simulink model "adcs_v14_speed"  (Simulink 7.4)
settings: Solver=ode4  StartTime=0.0  StopTime=80000  FixedStep=s_SIM_STEP_SIZE  RelTol=1e-3
values from neighbouring files (symbols this model uses):
  A = ((T_SIDE + .29)*1e-3)^2    [constants_v13.m]    (also in constants_v15.m; constants_v15_Pow.m; constants_v15_Pow_ss_error.m; constants_v16_integral_kartavya.m)
  Ca_Solar_Drag = 1.4    [constants_v13.m]    (also in constants_v15.m = 0; constants_v15_Pow.m; constants_v15_Pow_ss_error.m; constants_v16_integral_kartavya.m)
  Cd = 2.2    [constants_v13.m]    (also in constants_v15.m = 0; constants_v15_Pow.m; constants_v15_Pow_ss_error.m; constants_v16_integral_kartavya.m)
  check_time = 60000    [constants_v13.m]    (also in constants_v15.m = 10000; constants_v15_Pow_ss_error.m = 10000; constants_v16_integral_kartavya.m = 10000; constants_v16_integral_light_sun_sgp_igrf_power_13Dec2011.m = 10000)
  I_MAX = 0.5    [constants_v13.m]    (also in constants_v15.m; constants_v15_Pow.m; constants_v15_Pow_ss_error.m; constants_v16_integral_kartavya.m)
  I_TORQUER = 3.6 / 7.31    (= 0.492476060192)    [constants_v13.m]    (also in constants_v15.m = 0.272727272727; constants_v15_Pow.m; constants_v15_Pow_ss_error.m; constants_v16_integral_kartavya.m)
  Kd = 2* m_INERTIA / (s_numOrbits * T_ORBIT )    [constants_v13.m]    (also in constants_v15.m = m_INERTIA * (2 + delta)* zeta * w; constants_v15_Pow.m = m_INERTIA * (2 + delta)* zeta * w; constants_v15_Pow_ss_error.m = m_INERTIA * (2 + delta)* zeta * w; constants_v16_integral_kartavya.m = m_INERTIA * (2 + delta)* zeta * w)
  Kdetumb = K_det*eye(3)    [constants_v13.m]    (also in constants_v15.m; constants_v15_Pow.m; constants_v15_Pow_ss_error.m; constants_v16_integral_kartavya.m)
  Kp = m_INERTIA / (s_numOrbits * T_ORBIT * zeta)^2    [constants_v13.m]    (also in constants_v15.m = m_INERTIA * (w*w + 2*delta*zeta^2*w^2); constants_v15_Pow.m = m_INERTIA * (w*w + 2*delta*zeta^2*w^2); constants_v15_Pow_ss_error.m = m_INERTIA * (w*w + 2*delta*zeta^2*w^2); constants_v16_integral_kartavya.m = m_INERTIA * (w*w + 2*delta*zeta^2*w^2))
  m_INERTIA = [Ixx Ixy Ixz; Ixy Iyy Iyz; Ixz Iyz Izz]    [constants_v13.m]    (also in constants_v15.m; constants_v15_Pow.m = 1*[Ixx Ixy Ixz; Ixy Iyy Iyz; Ixz Iyz Izz]; constants_v15_Pow_ss_error.m = 1*[Ixx Ixy Ixz; Ixy Iyy Iyz; Ixz Iyz Izz]; constants_v16_integral_kartavya.m)
  mu = 6.673e-11*5.9742e24    (= 398658366000000)    [constants_v13.m]    (also in constants_v15.m; constants_v15_Pow.m; constants_v15_Pow_ss_error.m; constants_v16_integral_kartavya.m)
  N = 40    [constants_v13.m]    (also in constants_v15.m = 60; constants_v15_Pow.m; constants_v15_Pow_ss_error.m; constants_v16_integral_kartavya.m)
  P_momentum_flux_from_the_sun = 4.4e-6    (= 4.4e-06)    [constants_v13.m]    (also in constants_v15.m = 0; constants_v15_Pow.m; constants_v15_Pow_ss_error.m; constants_v16_integral_kartavya.m)
  q_BI0 = x_fromEnvModel(1:4)'    [OILS_script.m]    (also in OILS_script_OBC_preflight_bounce_back.m; OILS_script_extended.m; OILS_script_preflight_test.m; constants_v13.m = euler2qBI(roll0,pitch0,yaw0))
  s_FRAME_SIZE = 2    [constants_v13.m]    (also in constants_v15.m; constants_v15_Pow.m; constants_v15_Pow_ss_error.m; constants_v16_integral_kartavya.m)
  s_m_MAX = 0.95    [constants_v13.m]    (also in constants_v15.m; constants_v15_Pow.m; constants_v15_Pow_ss_error.m; constants_v16_integral_kartavya.m)
  s_MAG_B = 2.5e-5    (= 2.5e-05)    [constants_v13.m]    (also in constants_v15.m; constants_v15_Pow.m; constants_v15_Pow_ss_error.m; constants_v16_integral_kartavya.m)
  s_MAGMETER_WEIGHT = .9    (= 0.9)    [constants_v13.m]    (also in constants_v15.m; constants_v15_Pow.m; constants_v15_Pow_ss_error.m; constants_v16_integral_kartavya.m)
  s_SIM_STEP_SIZE = 0.1    [constants_v13.m]    (also in constants_v15.m; constants_v15_Pow.m; constants_v15_Pow_ss_error.m; constants_v16_integral_kartavya.m)
  s_SS_ADC_gain = 5    [constants_v13.m]    (also in constants_v15.m = 3.3; constants_v15_Pow.m; constants_v15_Pow_ss_error.m; constants_v16_integral_kartavya.m)
  s_SS_ADC_res = 2^12 - 1    (= 4095)    [constants_v13.m]    (also in constants_v15.m = 1023; constants_v15_Pow.m; constants_v15_Pow_ss_error.m; constants_v16_integral_kartavya.m)
  s_SS_MAX_ANGLE = 85    [constants_v13.m]    (also in constants_v15.m = 55; constants_v15_Pow.m; constants_v15_Pow_ss_error.m; constants_v16_integral_kartavya.m)
  s_TAU_W = 60    [constants_v13.m]    (also in constants_v15.m; constants_v15_Pow.m; constants_v15_Pow_ss_error.m; constants_v16_integral_kartavya.m)
  s_x_MAGMETER_BIAS = 50e-9    (= 5e-08)    [constants_v13.m]    (also in constants_v15.m = 0; constants_v15_Pow.m; constants_v15_Pow_ss_error.m; constants_v16_integral_kartavya.m)
  side = 0.26    [constants_v13.m]    (also in constants_v15.m; constants_v15_Pow.m; constants_v15_Pow_ss_error.m; constants_v16_integral_kartavya.m)
  Snum = 6    [constants_v13.m]    (also in constants_v15.m; constants_v15_Pow.m; constants_v15_Pow_ss_error.m; constants_v16_integral_kartavya.m)
  tol_q4 = 0.7    [constants_v13.m]    (also in constants_v15.m = 0.85; constants_v15_Pow.m = 0.85; constants_v15_Pow_ss_error.m = 0.85; constants_v16_integral_kartavya.m = 0.85)
  tol_w = 4e-3    (= 0.004)    [constants_v13.m]    (also in constants_v15.m; constants_v15_Pow.m; constants_v15_Pow_ss_error.m; constants_v16_integral_kartavya.m)
  Ts_display = 6    [constants_v13.m]    (also in constants_v15.m = 2; constants_v15_Pow.m; constants_v15_Pow_ss_error.m; constants_v16_integral_kartavya.m)
  v_COM_to_COP_b = [.2; 1.75; .2]*1e-2    [constants_v13.m]    (also in constants_v15.m = [.2; 1.75; .2]*0e-2; constants_v15_Pow.m; constants_v15_Pow_ss_error.m; constants_v16_integral_kartavya.m)
  v_S1 = [1 0 0]    [constants_v13.m]    (also in constants_v15.m; constants_v15_Pow.m; constants_v15_Pow_ss_error.m; constants_v16_integral_kartavya.m)
  v_S2 = [-1 0 0]    [constants_v13.m]    (also in constants_v15.m; constants_v15_Pow.m; constants_v15_Pow_ss_error.m; constants_v16_integral_kartavya.m)
  v_S3 = [0 1 0]    [constants_v13.m]    (also in constants_v15.m; constants_v15_Pow.m; constants_v15_Pow_ss_error.m; constants_v16_integral_kartavya.m)
  v_S4 = [0 -1 0]    [constants_v13.m]    (also in constants_v15.m; constants_v15_Pow.m; constants_v15_Pow_ss_error.m; constants_v16_integral_kartavya.m)
  v_S5 = [0 0 1]    [constants_v13.m]    (also in constants_v15.m; constants_v15_Pow.m; constants_v15_Pow_ss_error.m; constants_v16_integral_kartavya.m)
  v_S6 = [0 0 -1]    [constants_v13.m]    (also in constants_v15.m; constants_v15_Pow.m; constants_v15_Pow_ss_error.m; constants_v16_integral_kartavya.m)
  v_x_MOUNTING_THETA_ZYX_BODY_TORQUER = [1; 1; 1]* pi/180    [constants_v13.m]    (also in constants_v15.m; constants_v15_Pow.m; constants_v15_Pow_ss_error.m; constants_v16_integral_kartavya.m)
  wx0 = x_fromEnvModel(5)    [OILS_script.m]    (also in OILS_script_OBC_preflight_bounce_back.m; OILS_script_extended.m; OILS_script_preflight_test.m; constants_v13.m = 0.0349065850399)
  wy0 = x_fromEnvModel(6)    [OILS_script.m]    (also in OILS_script_OBC_preflight_bounce_back.m; OILS_script_extended.m; OILS_script_preflight_test.m; constants_v13.m = 0.0174532925199)
  wz0 = x_fromEnvModel(7)    [OILS_script.m]    (also in OILS_script_OBC_preflight_bounce_back.m; OILS_script_extended.m; OILS_script_preflight_test.m; constants_v13.m = -0.0349065850399)
libraries: commnoisgen2 x7, simulink x4, aerolibutil x2
(part 1 of 2)
settings Model: Creator=Jaideep  LastModifiedBy=Jaideep  SimulationMode=rapid-accelerator  ExtModeTrigDuration=100
settings SolverCC: AutoInsertRateTranBlk=on
settings DataIOCC: SaveFinalState=on  SaveOutput=off  SaveState=on  StateSaveName=tmp_raccel_xout
settings OptimizationCC: EfficientMapNaN2IntZero=off
settings HardwareCC: TargetEndianess=LittleEndian  TargetHWDeviceType=MATLAB Host  ProdEqTarget=off
settings RTWCC: SystemTargetFile=raccel.tlc  TemplateMakefile=raccel_default_tmf  RTWVerbose=off  ProcessScript=raccel_make_rtw_hook
settings CodeAppCC: GenerateComments=off  MaxIdLength=128  SimulinkBlockComments=off
settings RaccelTargetCC: TargetFunctionLibrary=ANSI_C  ERTMultiwordTypeDef=System defined  ERTMultiwordLength=256  IsPILTarget=off  ParMdlRefBuildCompliant=off  GeneratePreprocessorConditionals=Disable all  ERTFirstTimeCompliant=off  MultiInstanceERTCode=off  EnableShiftOperators=on  PortableWordSizes=off  RTWCAPISignals=off  RTWCAPIParams=off

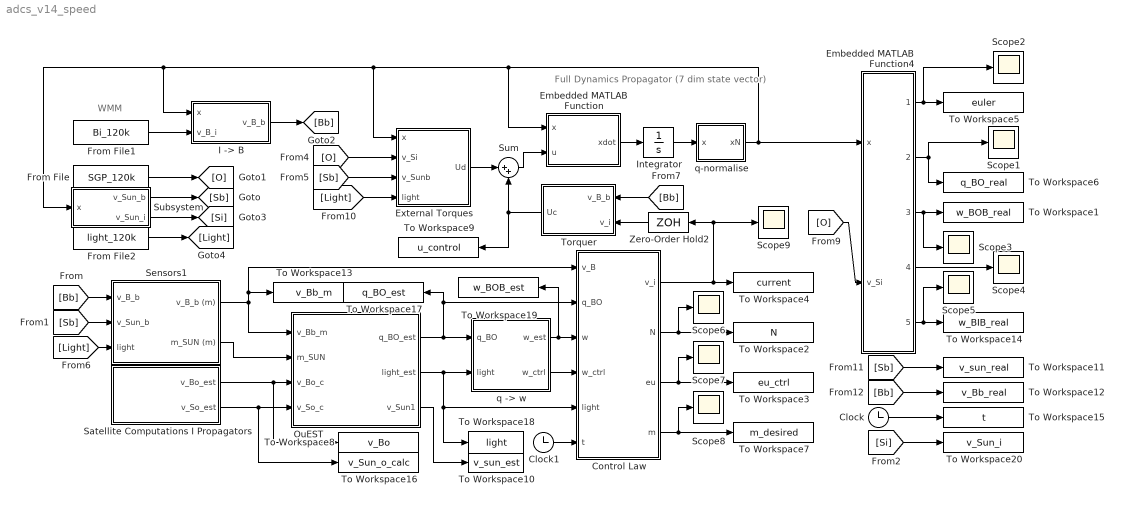
== system adcs_v14_speed ==
  note: Full Dynamics Propagator
      |  (7 dim state vector)
  note: WMM
  Clock : Clock
      settings: Decimation=10
  Clock1 : Clock
      settings: Decimation=10
  Control Law : Subsystem  TreatAsAtomicUnit=on  SystemSampleTime=s_FRAME_SIZE
  Embedded MATLAB Function : Stateflow chart
  Embedded MATLAB Function4 : Stateflow chart
  External Torques : Subsystem
  From File : FromFile  FileName=SGP_120k
  From File1 : FromFile  FileName=Bi_120k
  From File2 : FromFile  FileName=light_120k  SampleTime=0
  "I -> B" : Subsystem
  Integrator : Integrator  InitialCondition=[q_BI0; wx0; wy0; wz0]
  QuEST : Stateflow chart  TreatAsAtomicUnit=on  SystemSampleTime=s_FRAME_SIZE
  Satellite Computations I Propagators : Subsystem  TreatAsAtomicUnit=on  SystemSampleTime=s_FRAME_SIZE
  Scope{1..9} (9 alike) : Scope
      Scope1 settings: YMin=-10  YMax=10  SaveName=ScopeData11  SampleInput=on  SampleTime=Ts_display
      Scope2 settings: TimeRange=80000  YMin=-70  YMax=60  SaveName=ScopeData7  SampleInput=on  SampleTime=Ts_display
      Scope3 settings: YMin=-10  YMax=10  SaveName=ScopeData13  SampleInput=on  SampleTime=Ts_display
      Scope4 settings: YMin=-10  YMax=10  SaveName=ScopeData14  SampleInput=on  SampleTime=Ts_display
      Scope5 settings: YMin=-10  YMax=10  SaveName=ScopeData15  SampleInput=on  SampleTime=Ts_display
      Scope6 settings: YMin=-10  YMax=10  SaveName=ScopeData16  SampleInput=on  SampleTime=Ts_display
      Scope7 settings: YMin=-10  YMax=10  SaveName=ScopeData20  SampleInput=on  SampleTime=Ts_display
      Scope8 settings: YMin=-10  YMax=10  SaveName=ScopeData21  SampleInput=on  SampleTime=Ts_display
      Scope9 settings: YMin=-10  YMax=10  SaveName=ScopeData23  SampleInput=on  SampleTime=Ts_display
  Sensors1 : Subsystem
  Subsystem : Subsystem
  Sum : Sum  Inputs=|++  OutDataType=sfix(16)  OutScaling=2^0
  To Workspace1 : ToWorkspace  VariableName=w_BOB_real  SampleTime=Ts_display  SaveFormat=Array
  To Workspace10 : ToWorkspace  VariableName=v_sun_est  SampleTime=Ts_display  SaveFormat=Array
  To Workspace11 : ToWorkspace  VariableName=v_sun_real  SampleTime=Ts_display  SaveFormat=Array
  To Workspace12 : ToWorkspace  VariableName=v_Bb_real  SampleTime=Ts_display  SaveFormat=Array
  To Workspace13 : ToWorkspace  VariableName=v_Bb_m  SampleTime=Ts_display  SaveFormat=Array
  To Workspace14 : ToWorkspace  VariableName=w_BIB_real  SampleTime=Ts_display  SaveFormat=Array
  To Workspace15 : ToWorkspace  VariableName=t  SampleTime=Ts_display  SaveFormat=Array
  To Workspace16 : ToWorkspace  VariableName=v_Sun_o_calc  SampleTime=Ts_display  SaveFormat=Array
  To Workspace17 : ToWorkspace  VariableName=q_BO_est  SampleTime=Ts_display  SaveFormat=Array
  To Workspace18 : ToWorkspace  VariableName=light  SampleTime=Ts_display  SaveFormat=Array
  To Workspace19 : ToWorkspace  VariableName=w_BOB_est  SampleTime=Ts_display  SaveFormat=Array
  To Workspace2 : ToWorkspace  VariableName=N  SampleTime=Ts_display  SaveFormat=Array
  To Workspace20 : ToWorkspace  VariableName=v_Sun_i  SampleTime=Ts_display  SaveFormat=Array
  To Workspace3 : ToWorkspace  VariableName=eu_ctrl  SampleTime=Ts_display  SaveFormat=Array
  To Workspace4 : ToWorkspace  VariableName=current  SampleTime=Ts_display  SaveFormat=Array
  To Workspace5 : ToWorkspace  VariableName=euler  SampleTime=Ts_display  SaveFormat=Array
  To Workspace6 : ToWorkspace  VariableName=q_BO_real  SampleTime=Ts_display  SaveFormat=Array
  To Workspace7 : ToWorkspace  VariableName=m_desired  SampleTime=Ts_display  SaveFormat=Array
  To Workspace8 : ToWorkspace  VariableName=v_Bo  SampleTime=Ts_display  SaveFormat=Array
  To Workspace9 : ToWorkspace  VariableName=u_control  SampleTime=Ts_display  SaveFormat=Array
  Torquer : Subsystem
  Zero-Order Hold2 : ZeroOrderHold  SampleTime=s_FRAME_SIZE
  "q -> w" : Subsystem  TreatAsAtomicUnit=on  SystemSampleTime=s_FRAME_SIZE
  q-normalise : Stateflow chart
  wires:
  Embedded MATLAB Function/1(xdot) -> Integrator/1
  Integrator/1 -> q-normalise/1(x)
  From File/1 -> [O]
  q-normalise/1(xN) -> Subsystem/1(x), "I -> B"/1(x), External Torques/1(x), Embedded MATLAB Function/1(x), Embedded MATLAB Function4/1(x)
  Sum/1 -> Embedded MATLAB Function/2(u)
  "I -> B"/1(v_B_b) -> [Bb]
  Subsystem/1(v_Sun_b) -> [Sb]
  [Bb] -> Sensors1/1(v_B_b)
  [Sb] -> Sensors1/2(v_Sun_b)
  Subsystem/2(v_Sun_i) -> [Si]
  [O] -> External Torques/2(v_Si)
  [Sb] -> External Torques/3(v_Sunb)
  [Bb] -> Torquer/1(v_B_b)
  [Light] -> Sensors1/3(light)
  Sensors1/2(m_SUN (m)) -> QuEST/2(m_SUN)
  Sensors1/1(v_B_b (m)) -> QuEST/1(v_Bb_m), Control Law/1(v_B), To Workspace13/1
  Zero-Order Hold2/1 -> Torquer/2(v_i)
  External Torques/1(Ud) -> Sum/1
  Torquer/1(Uc) -> Sum/2, To Workspace9/1
  Satellite Computations I Propagators/1(v_Bo_est) -> To Workspace8/1, QuEST/3(v_Bo_c)
  Satellite Computations I Propagators/2(v_So_est) -> To Workspace16/1, QuEST/4(v_So_c)
  QuEST/1(q_BO_est) -> "q -> w"/1(q_BO), Control Law/2(q_BO), To Workspace17/1
  QuEST/2(light_est) -> "q -> w"/2(light), Control Law/5(light), To Workspace18/1
  Control Law/1(v_i) -> To Workspace4/1, Zero-Order Hold2/1, Scope9/1
  [O] -> Embedded MATLAB Function4/2(v_Si)
  Control Law/2(N) -> To Workspace2/1, Scope6/1
  From File2/1 -> [Light]
  Control Law/3(eu) -> To Workspace3/1, Scope7/1
  Control Law/4(m) -> To Workspace7/1, Scope8/1
  "q -> w"/1(w_est) -> Control Law/3(w), To Workspace19/1
  [Light] -> External Torques/4(light)
  "q -> w"/2(w_ctrl) -> Control Law/4(w_ctrl)
  QuEST/3(v_Sun1) -> To Workspace10/1
  [Sb] -> To Workspace11/1
  [Bb] -> To Workspace12/1
  Clock/1 -> To Workspace15/1
  From File1/1 -> "I -> B"/2(v_B_i)
  Clock1/1 -> Control Law/6(t)
  Embedded MATLAB Function4/3(w_BOB) -> To Workspace1/1, Scope3/1
  Embedded MATLAB Function4/2(q_BO) -> To Workspace6/1, Scope1/1
  Embedded MATLAB Function4/1(euler) -> To Workspace5/1, Scope2/1
  Embedded MATLAB Function4/5(w_BIB) -> To Workspace14/1, Scope5/1
  Embedded MATLAB Function4/4(modw) -> Scope4/1
  [Si] -> To Workspace20/1

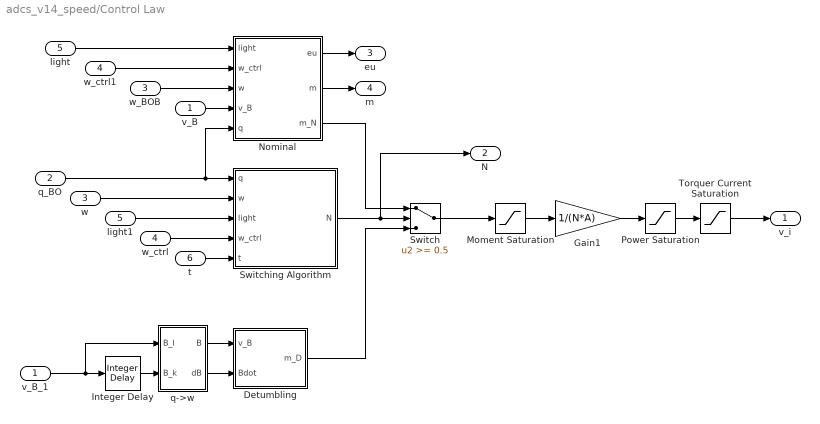
== system adcs_v14_speed/Control Law ==
  v_B : Inport  OutDataType=sfix(16)  OutScaling=2^0
  q_BO : Inport  Port=2  OutDataType=sfix(16)  OutScaling=2^0
  w : Inport  Port=3  OutDataType=sfix(16)  OutScaling=2^0
  w_ctrl : Inport  Port=4  OutDataType=sfix(16)  OutScaling=2^0
  light : Inport  Port=5  OutDataType=sfix(16)  OutScaling=2^0
  t : Inport  Port=6  OutDataType=sfix(16)  OutScaling=2^0
  Detumbling : Stateflow chart
  Gain1 : Gain  Gain=1/(N*A)  ParameterDataType=sfix(16)  ParameterScaling=2^0  OutDataType=sfix(16)  OutScaling=2^0
  Integer Delay : simulink/Discrete/Integer Delay  vinit=0.0  samptime=-1  NumDelays=1
  Moment Saturation : Saturate  UpperLimit=s_m_MAX  LowerLimit=-s_m_MAX  OutDataType=sfix(16)  OutScaling=2^0
  Nominal : Stateflow chart
  Power Saturation : Saturate  UpperLimit=I_MAX  LowerLimit=-I_MAX  OutDataType=sfix(16)  OutScaling=2^0
  Switch : Switch  Threshold=0.5  OutDataType=sfix(16)  OutScaling=2^0
  Switching Algorithm : Subsystem
  Torquer Current Saturation : Saturate  UpperLimit=I_TORQUER  LowerLimit=-I_TORQUER  OutDataType=sfix(16)  OutScaling=2^0
  light1 : InportShadow  Port=5  OutDataType=sfix(16)  OutScaling=2^0  LatchByCopyingInsideSignal=off
  q->w : Stateflow chart
  v_B_1 : InportShadow  Port=1  OutDataType=sfix(16)  OutScaling=2^0  LatchByCopyingInsideSignal=off
  w_BOB : InportShadow  Port=3  OutDataType=sfix(16)  OutScaling=2^0  LatchByCopyingInsideSignal=off
  w_ctrl1 : InportShadow  Port=4  OutDataType=sfix(16)  OutScaling=2^0  LatchByCopyingInsideSignal=off
  v_i : Outport  OutDataType=sfix(16)  OutScaling=2^0
  N : Outport  Port=2  OutDataType=sfix(16)  OutScaling=2^0
  eu : Outport  Port=3  OutDataType=sfix(16)  OutScaling=2^0
  m : Outport  Port=4  OutDataType=sfix(16)  OutScaling=2^0
  wires:
  w_ctrl/1 -> Switching Algorithm/4(w_ctrl)
  Nominal/2(m) -> m/1
  Nominal/1(eu) -> eu/1
  w_BOB/1 -> Nominal/3(w)
  light1/1 -> Switching Algorithm/3(light)
  v_B/1 -> Nominal/4(v_B)
  q->w/2(dB) -> Detumbling/2(Bdot)
  v_B_1/1 -> Integer Delay/1, q->w/1(B_l)
  w/1 -> Switching Algorithm/2(w)
  Nominal/3(m_N) -> Switch/1
  Switching Algorithm/1(N) -> Switch/2, N/1
  Detumbling/1(m_D) -> Switch/3
  Switch/1 -> Moment Saturation/1
  Power Saturation/1 -> Torquer Current Saturation/1
  Moment Saturation/1 -> Gain1/1
  Torquer Current Saturation/1 -> v_i/1
  Gain1/1 -> Power Saturation/1
  light/1 -> Nominal/1(light)
  q_BO/1 -> Switching Algorithm/1(q), Nominal/5(q)
  Integer Delay/1 -> q->w/2(B_k)
  q->w/1(B) -> Detumbling/1(v_B)
  t/1 -> Switching Algorithm/5(t)
  w_ctrl1/1 -> Nominal/2(w_ctrl)

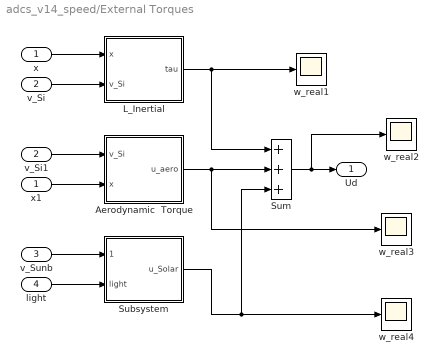
== system adcs_v14_speed/External Torques ==
  x : Inport  OutDataType=sfix(16)  OutScaling=2^0
  v_Si : Inport  Port=2  OutDataType=sfix(16)  OutScaling=2^0
  v_Sunb : Inport  Port=3  OutDataType=sfix(16)  OutScaling=2^0
  light : Inport  Port=4  OutDataType=sfix(16)  OutScaling=2^0
  Aerodynamic  Torque : Subsystem
  L_Inertial : Stateflow chart
  Subsystem : Subsystem
  Sum : Sum  Inputs=+++  OutDataType=fixdt(1, 16)  OutScaling=2^0
  v_Si1 : InportShadow  Port=2  OutDataType=sfix(16)  OutScaling=2^0  LatchByCopyingInsideSignal=off
  w_real{1..4} (4 alike) : Scope
      w_real1 settings: TimeRange=80000  YMin=-3e-009  YMax=1.1e-008  SaveName=ScopeData18  SampleInput=on  SampleTime=5
      w_real2 settings: TimeRange=80000  YMin=-7e-009  YMax=1e-008  SaveName=ScopeData17  SampleInput=on  SampleTime=5
      w_real3 settings: YMin=-8e-010  YMax=1.4e-009  SaveName=ScopeData19  SampleInput=on  SampleTime=5
      w_real4 settings: YMin=-6e-009  YMax=1e-008  SaveName=ScopeData22  SampleInput=on  SampleTime=5
  x1 : InportShadow  Port=1  OutDataType=sfix(16)  OutScaling=2^0  LatchByCopyingInsideSignal=off
  Ud : Outport  OutDataType=sfix(16)  OutScaling=2^0
  wires:
  x/1 -> L_Inertial/1(x)
  v_Si/1 -> L_Inertial/2(v_Si)
  L_Inertial/1(tau) -> Sum/1, w_real1/1
  Aerodynamic  Torque/1(u_aero) -> Sum/2, w_real3/1
  x1/1 -> Aerodynamic  Torque/2(x)
  v_Si1/1 -> Aerodynamic  Torque/1(v_Si)
  Sum/1 -> Ud/1, w_real2/1
  v_Sunb/1 -> Subsystem/1(v_Sun_b)
  Subsystem/1(u_Solar) -> Sum/3, w_real4/1
  light/1 -> Subsystem/2(light)

== system adcs_v14_speed/I -> B ==
  x : Inport  OutDataType=sfix(16)  OutScaling=2^0
  v_B_i : Inport  Port=2  OutDataType=sfix(16)  OutScaling=2^0
  Gain : Gain  Gain=1e-9  ParameterDataType=fixdt(1, 16)  ParameterScaling=2^0  OutDataType=fixdt(1, 16)  OutScaling=2^0
  L_Inertial : Stateflow chart
  v_B_b : Outport  OutDataType=sfix(16)  OutScaling=2^0
  wires:
  L_Inertial/1(v_B) -> v_B_b/1
  x/1 -> L_Inertial/1(x)
  v_B_i/1 -> Gain/1
  Gain/1 -> L_Inertial/2(v_I)

== system adcs_v14_speed/Satellite Computations I Propagators ==
  From File : FromFile  FileName=Si_120k
  From File2 : FromFile  FileName=SGP_est_120k
  From File3 : FromFile  FileName=Bi8_est_120k
  m_TOI_NEW : Stateflow chart
  m_TOI_NEW1 : Stateflow chart
  v_Bo_est : Outport  OutDataType=sfix(16)  OutScaling=2^0
  v_So_est : Outport  Port=2  OutDataType=sfix(16)  OutScaling=2^0
  wires:
  From File3/1 -> m_TOI_NEW/2(v_I)
  From File2/1 -> m_TOI_NEW1/2(ECI), m_TOI_NEW/1(ECI)
  From File/1 -> m_TOI_NEW1/1(v_I)
  m_TOI_NEW/1(v_O) -> v_Bo_est/1
  m_TOI_NEW1/1(v_O) -> v_So_est/1

== system adcs_v14_speed/Sensors1 ==
  note: 'm' stands for measured
  v_B_b : Inport  OutDataType=sfix(16)  OutScaling=2^0
  v_Sun_b : Inport  Port=2  OutDataType=sfix(16)  OutScaling=2^0
  light : Inport  Port=3  OutDataType=sfix(16)  OutScaling=2^0
  Magnetometer simple : Subsystem
  Sun Sensors : Subsystem
  v_B_b (m) : Outport  OutDataType=sfix(16)  OutScaling=2^0
  m_SUN (m) : Outport  Port=2  OutDataType=sfix(16)  OutScaling=2^0
  wires:
  light/1 -> Sun Sensors/2(Light)
  Magnetometer simple/1(v_B_b(m)) -> v_B_b (m)/1
  v_B_b/1 -> Magnetometer simple/1(v_B_b)
  v_Sun_b/1 -> Sun Sensors/1(v_Sun_b)
  Sun Sensors/1(m_SUN) -> m_SUN (m)/1

== system adcs_v14_speed/Subsystem ==
  x : Inport  OutDataType=sfix(16)  OutScaling=2^0
  From File : FromFile  FileName=Si_120k  SampleTime=0
  f: I->B : Stateflow chart
  v_Sun_b : Outport  OutDataType=sfix(16)  OutScaling=2^0
  v_Sun_i : Outport  Port=2  OutDataType=sfix(16)  OutScaling=2^0
  wires:
  x/1 -> f: I->B/1(x)
  f: I->B/1(v_B) -> v_Sun_b/1
  From File/1 -> f: I->B/2(v_I), v_Sun_i/1

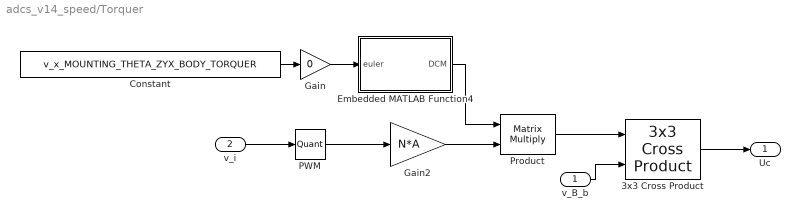
== system adcs_v14_speed/Torquer ==
  v_B_b : Inport  OutDataType=sfix(16)  OutScaling=2^0
  v_i : Inport  Port=2  OutDataType=sfix(16)  OutScaling=2^0
  3x3 Cross Product : aerolibutil/3x3 Cross Product  SystemSampleTime=-1
  Constant : Constant  Value=v_x_MOUNTING_THETA_ZYX_BODY_TORQUER  OutDataType=sfix(16)  OutScaling=2^0
  Embedded MATLAB Function4 : Stateflow chart
  Gain : Gain  Gain=0  ParameterDataType=sfix(16)  ParameterScaling=2^0  OutDataType=sfix(16)  OutScaling=2^0
  Gain2 : Gain  Gain=N*A  ParameterDataType=sfix(16)  ParameterScaling=2^0  OutDataType=sfix(16)  OutScaling=2^0
  PWM : Quantizer  QuantizationInterval=s_PWM_RES
  Product : Product  Multiplication=Matrix(*)  OutDataType=sfix(16)  OutScaling=2^0  RndMeth=Zero
  Uc : Outport  OutDataType=sfix(16)  OutScaling=2^0
  wires:
  PWM/1 -> Gain2/1
  v_B_b/1 -> 3x3 Cross Product/2
  3x3 Cross Product/1 -> Uc/1
  v_i/1 -> PWM/1
  Embedded MATLAB Function4/1(DCM) -> Product/1
  Gain2/1 -> Product/2
  Product/1 -> 3x3 Cross Product/1
  Constant/1 -> Gain/1
  Gain/1 -> Embedded MATLAB Function4/1(euler)

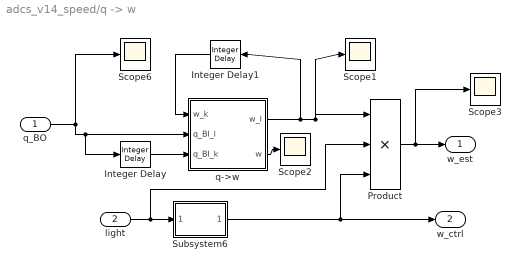
== system adcs_v14_speed/q -> w ==
  q_BO : Inport
  light : Inport  Port=2
  Integer Delay : simulink/Discrete/Integer Delay  vinit=0.0  samptime=-1  NumDelays=1
  Integer Delay1 : simulink/Discrete/Integer Delay  vinit=[0;0;0]  samptime=-1  NumDelays=1
  Product : Product  Inputs=3  OutDataType=fixdt(1, 16)  OutScaling=2^0  RndMeth=Zero
  Scope{1..3,6} (4 alike) : Scope
      Scope1 settings: YMin=-10  YMax=10  SaveName=ScopeData9  SampleInput=on
      Scope2 settings: YMin=-10  YMax=10  SaveName=ScopeData10  SampleInput=on
      Scope3 settings: YMin=-10  YMax=10  SaveName=ScopeData12  SampleInput=on
      Scope6 settings: YMin=-10  YMax=10  SaveName=ScopeData8  SampleInput=on
  Subsystem6 : Subsystem
  q->w : Stateflow chart
  w_est : Outport
  w_ctrl : Outport  Port=2
  wires:
  Subsystem6/1(w-ctrl) -> w_ctrl/1, Product/3
  q_BO/1 -> Integer Delay/1, q->w/2(q_BI_l), Scope6/1
  light/1 -> Product/2, Subsystem6/1(light)
  Product/1 -> w_est/1, Scope3/1
  Integer Delay/1 -> q->w/3(q_BI_k)
  q->w/1(w_l) -> Integer Delay1/1, Product/1, Scope1/1
  Integer Delay1/1 -> q->w/1(w_k)
  q->w/2(w) -> Scope2/1

== system adcs_v14_speed/Control Law/Switching Algorithm ==
  note: remov the t=0 checking
      | code, not necessary
  q : Inport  OutDataType=sfix(16)  OutScaling=2^0
  w : Inport  Port=2  OutDataType=sfix(16)  OutScaling=2^0
  light : Inport  Port=3  OutDataType=sfix(16)  OutScaling=2^0
  w_ctrl : Inport  Port=4  OutDataType=sfix(16)  OutScaling=2^0
  t : Inport  Port=5  OutDataType=sfix(16)  OutScaling=2^0
  Unit Delay : UnitDelay  SampleTime=-1
  gate pulse : Stateflow chart
  N : Outport  OutDataType=sfix(16)  OutScaling=2^0
  wires:
  t/1 -> gate pulse/3(t)
  w_ctrl/1 -> gate pulse/5(w_ctrl)
  light/1 -> gate pulse/4(light_flag)
  gate pulse/1(N) -> N/1
  q/1 -> gate pulse/2(q)
  Unit Delay/1 -> gate pulse/6(time2)
  gate pulse/2(time1) -> Unit Delay/1
  w/1 -> gate pulse/1(w)

== system adcs_v14_speed/External Torques/Aerodynamic  Torque ==
  v_Si : Inport
  x : Inport  Port=2
  Demux : Demux  Outputs=2
  aero torque : Stateflow chart
  v_I to v_B : Stateflow chart
  u_aero : Outport  OutDataType=sfix(16)  OutScaling=2^0
  wires:
  v_I to v_B/1(v_B) -> aero torque/2(v_B)
  v_Si/1 -> Demux/1
  Demux/2 -> v_I to v_B/1(v_I)
  x/1 -> v_I to v_B/2(x)
  aero torque/1(u_aero) -> u_aero/1

== system adcs_v14_speed/External Torques/Subsystem ==
  v_Sun_b : Inport  OutDataType=sfix(16)  OutScaling=2^0
  light : Inport  Port=2  OutDataType=sfix(16)  OutScaling=2^0
  Solar_drag : Stateflow chart
  Vector from CoM to CoP_in Body frame (yet to be finalized)2 : Constant  Value=v_COM_to_COP_b  VectorParams1D=off  OutDataType=sfix(16)  OutScaling=2^0
  _ : aerolibutil/3x3 Cross Product  SystemSampleTime=-1
  u_Solar : Outport  OutDataType=sfix(16)  OutScaling=2^0
  wires:
  _/1 -> u_Solar/1
  v_Sun_b/1 -> Solar_drag/1(v_Sun_b)
  light/1 -> Solar_drag/2(light)
  Solar_drag/1(solar_drag) -> _/2
  Vector from CoM to CoP_in Body frame (yet to be finalized)2/1 -> _/1

== system adcs_v14_speed/Sensors1/Magnetometer simple ==
  v_B_b : Inport  OutDataType=sfix(16)  OutScaling=2^0
  Constant : Constant  Value=s_x_MAGMETER_BIAS  OutDataType=fixdt(1, 16)  OutScaling=2^0
  Gaussian Noise Generator : commnoisgen2/Gaussian Noise Generator  SystemSampleTime=-1  m=0  d=s_x_MAGMETER  s=41  Ts=s_SIM_STEP_SIZE  frameBased=off  sampPerFrame=1  orient=off  outDataType=double
  Sum1 : Sum  Inputs=+++  OutDataType=sfix(16)  OutScaling=2^0
  v_B_b(m) : Outport  OutDataType=sfix(16)  OutScaling=2^0
  wires:
  Constant/1 -> Sum1/3
  Sum1/1 -> v_B_b(m)/1
  Gaussian Noise Generator/1 -> Sum1/1
  v_B_b/1 -> Sum1/2

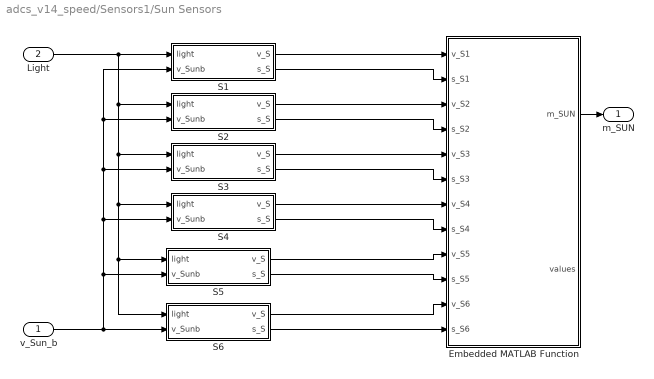
== system adcs_v14_speed/Sensors1/Sun Sensors ==
  v_Sun_b : Inport  OutDataType=sfix(16)  OutScaling=2^0
  Light : Inport  Port=2  OutDataType=sfix(16)  OutScaling=2^0
  Embedded MATLAB Function : Stateflow chart
  S1 : Subsystem
  S2 : Subsystem
  S3 : Subsystem
  S4 : Subsystem
  S5 : Subsystem
  S6 : Subsystem
  m_SUN : Outport  OutDataType=fixdt(1, 16)  OutScaling=2^0
  wires:
  Embedded MATLAB Function/1(m_SUN) -> m_SUN/1
  v_Sun_b/1 -> S6/2(v_Sunb), S5/2(v_Sunb), S4/2(v_Sunb), S3/2(v_Sunb), S2/2(v_Sunb), S1/2(v_Sunb)
  S1/1(v_S) -> Embedded MATLAB Function/1(v_S1)
  S1/2(s_S) -> Embedded MATLAB Function/2(s_S1)
  S2/1(v_S) -> Embedded MATLAB Function/3(v_S2)
  S2/2(s_S) -> Embedded MATLAB Function/4(s_S2)
  S3/1(v_S) -> Embedded MATLAB Function/5(v_S3)
  S3/2(s_S) -> Embedded MATLAB Function/6(s_S3)
  S4/1(v_S) -> Embedded MATLAB Function/7(v_S4)
  S4/2(s_S) -> Embedded MATLAB Function/8(s_S4)
  S5/1(v_S) -> Embedded MATLAB Function/9(v_S5)
  S5/2(s_S) -> Embedded MATLAB Function/10(s_S5)
  S6/1(v_S) -> Embedded MATLAB Function/11(v_S6)
  S6/2(s_S) -> Embedded MATLAB Function/12(s_S6)
  Light/1 -> S1/1(light), S2/1(light), S3/1(light), S4/1(light), S5/1(light), S6/1(light)

== system adcs_v14_speed/q -> w/Subsystem6 ==
  light : Inport  OutDataType=fixdt(1, 16)  OutScaling=2^0
  (1-L) + L/z : Stateflow chart
  Integer Delay : simulink/Discrete/Integer Delay  vinit=0.0  samptime=-1  NumDelays=300
  Scope : Scope
  Scope1 : Scope
  Scope2 : Scope
      settings: TimeRange=80000  SaveName=ScopeData2
  w-ctrl : Outport  OutDataType=fixdt(1, 16)  OutScaling=2^0
  wires:
  (1-L) + L/z/1(y) -> Scope/1, w-ctrl/1
  light/1 -> (1-L) + L/z/1(a), Integer Delay/1, Scope2/1
  Integer Delay/1 -> Scope1/1, (1-L) + L/z/2(b)

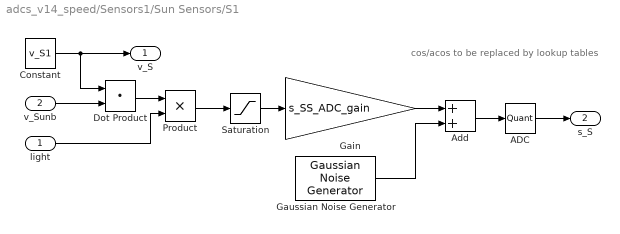
== system adcs_v14_speed/Sensors1/Sun Sensors/S1 ==
  note: cos/acos to be replaced by lookup tables
  light : Inport  OutDataType=sfix(16)  OutScaling=2^0
  v_Sunb : Inport  Port=2  OutDataType=sfix(16)  OutScaling=2^0
  ADC : Quantizer  QuantizationInterval=1/s_SS_ADC_res
  Add : Sum  OutDataType=sfix(16)  OutScaling=2^-10
  Constant : Constant  Value=v_S1  OutDataType=sfix(16)  OutScaling=2^0
  Dot Product : DotProduct  OutDataType=sfix(16)  OutScaling=2^-10  InputSameDT=on  OutDataTypeStr=Inherit: Inherit via internal rule
  Gain : Gain  Gain=s_SS_ADC_gain  ParameterDataType=sfix(16)  ParameterScaling=2^0  OutDataType=sfix(16)  OutScaling=2^0
  Gaussian Noise Generator : commnoisgen2/Gaussian Noise Generator  SystemSampleTime=-1  m=0  d=s_x_SUNSENSOR  s=41  Ts=s_SIM_STEP_SIZE  frameBased=off  sampPerFrame=1  orient=off  outDataType=double
  Product : Product  OutDataType=fixdt(1, 16)  OutScaling=2^0  RndMeth=Zero
  Saturation : Saturate  UpperLimit=inf  LowerLimit=0  OutDataType=sfix(16)  OutScaling=2^0
  v_S : Outport  OutDataType=sfix(16)  OutScaling=2^0
  s_S : Outport  Port=2  OutDataType=sfix(16)  OutScaling=2^0
  wires:
  light/1 -> Product/2
  Product/1 -> Saturation/1
  Dot Product/1 -> Product/1
  v_Sunb/1 -> Dot Product/2
  Saturation/1 -> Gain/1
  Constant/1 -> v_S/1, Dot Product/1
  Gaussian Noise Generator/1 -> Add/2
  Gain/1 -> Add/1
  Add/1 -> ADC/1
  ADC/1 -> s_S/1

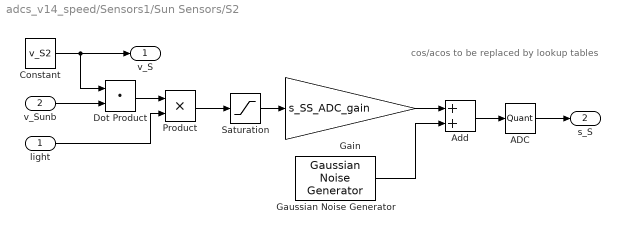
== system adcs_v14_speed/Sensors1/Sun Sensors/S2 ==
  note: cos/acos to be replaced by lookup tables
  light : Inport  OutDataType=sfix(16)  OutScaling=2^0
  v_Sunb : Inport  Port=2  OutDataType=sfix(16)  OutScaling=2^0
  ADC : Quantizer  QuantizationInterval=1/s_SS_ADC_res
  Add : Sum  OutDataType=sfix(16)  OutScaling=2^-10
  Constant : Constant  Value=v_S2  OutDataType=sfix(16)  OutScaling=2^0
  Dot Product : DotProduct  OutDataType=sfix(16)  OutScaling=2^-10  InputSameDT=on  OutDataTypeStr=Inherit: Inherit via internal rule
  Gain : Gain  Gain=s_SS_ADC_gain  ParameterDataType=sfix(16)  ParameterScaling=2^0  OutDataType=sfix(16)  OutScaling=2^0
  Gaussian Noise Generator : commnoisgen2/Gaussian Noise Generator  SystemSampleTime=-1  m=0  d=s_x_SUNSENSOR  s=41  Ts=s_SIM_STEP_SIZE  frameBased=off  sampPerFrame=1  orient=off  outDataType=double
  Product : Product  OutDataType=fixdt(1, 16)  OutScaling=2^0  RndMeth=Zero
  Saturation : Saturate  UpperLimit=inf  LowerLimit=0  OutDataType=sfix(16)  OutScaling=2^0
  v_S : Outport  OutDataType=sfix(16)  OutScaling=2^0
  s_S : Outport  Port=2  OutDataType=sfix(16)  OutScaling=2^0
  wires:
  ADC/1 -> s_S/1
  Add/1 -> ADC/1
  Gain/1 -> Add/1
  Gaussian Noise Generator/1 -> Add/2
  Constant/1 -> Dot Product/1, v_S/1
  Saturation/1 -> Gain/1
  v_Sunb/1 -> Dot Product/2
  Dot Product/1 -> Product/1
  Product/1 -> Saturation/1
  light/1 -> Product/2

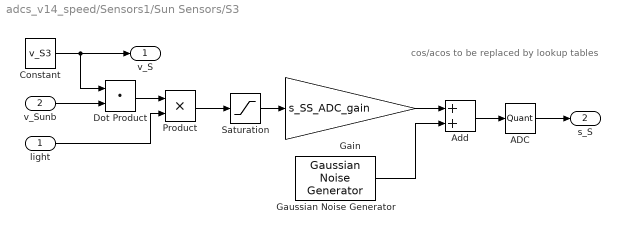
== system adcs_v14_speed/Sensors1/Sun Sensors/S3 ==
  note: cos/acos to be replaced by lookup tables
  light : Inport  OutDataType=sfix(16)  OutScaling=2^0
  v_Sunb : Inport  Port=2  OutDataType=sfix(16)  OutScaling=2^0
  ADC : Quantizer  QuantizationInterval=1/s_SS_ADC_res
  Add : Sum  OutDataType=sfix(16)  OutScaling=2^-10
  Constant : Constant  Value=v_S3  OutDataType=sfix(16)  OutScaling=2^0
  Dot Product : DotProduct  OutDataType=sfix(16)  OutScaling=2^-10  InputSameDT=on  OutDataTypeStr=Inherit: Inherit via internal rule
  Gain : Gain  Gain=s_SS_ADC_gain  ParameterDataType=sfix(16)  ParameterScaling=2^0  OutDataType=sfix(16)  OutScaling=2^0
  Gaussian Noise Generator : commnoisgen2/Gaussian Noise Generator  SystemSampleTime=-1  m=0  d=s_x_SUNSENSOR  s=41  Ts=s_SIM_STEP_SIZE  frameBased=off  sampPerFrame=1  orient=off  outDataType=double
  Product : Product  OutDataType=fixdt(1, 16)  OutScaling=2^0  RndMeth=Zero
  Saturation : Saturate  UpperLimit=inf  LowerLimit=0  OutDataType=sfix(16)  OutScaling=2^0
  v_S : Outport  OutDataType=sfix(16)  OutScaling=2^0
  s_S : Outport  Port=2  OutDataType=sfix(16)  OutScaling=2^0
  wires:
  light/1 -> Product/2
  Product/1 -> Saturation/1
  Dot Product/1 -> Product/1
  v_Sunb/1 -> Dot Product/2
  Saturation/1 -> Gain/1
  Constant/1 -> v_S/1, Dot Product/1
  Gaussian Noise Generator/1 -> Add/2
  Gain/1 -> Add/1
  Add/1 -> ADC/1
  ADC/1 -> s_S/1

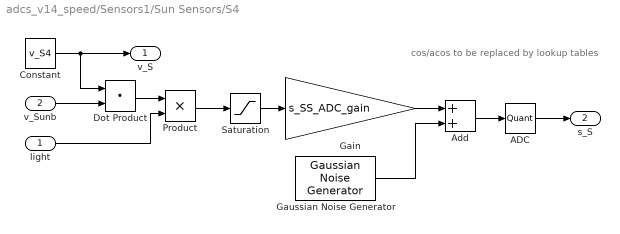
== system adcs_v14_speed/Sensors1/Sun Sensors/S4 ==
  note: cos/acos to be replaced by lookup tables
  light : Inport  OutDataType=sfix(16)  OutScaling=2^0
  v_Sunb : Inport  Port=2  OutDataType=sfix(16)  OutScaling=2^0
  ADC : Quantizer  QuantizationInterval=1/s_SS_ADC_res
  Add : Sum  OutDataType=sfix(16)  OutScaling=2^-10
  Constant : Constant  Value=v_S4  OutDataType=sfix(16)  OutScaling=2^0
  Dot Product : DotProduct  OutDataType=sfix(16)  OutScaling=2^-10  InputSameDT=on  OutDataTypeStr=Inherit: Inherit via internal rule
  Gain : Gain  Gain=s_SS_ADC_gain  ParameterDataType=sfix(16)  ParameterScaling=2^0  OutDataType=sfix(16)  OutScaling=2^0
  Gaussian Noise Generator : commnoisgen2/Gaussian Noise Generator  SystemSampleTime=-1  m=0  d=s_x_SUNSENSOR  s=41  Ts=s_SIM_STEP_SIZE  frameBased=off  sampPerFrame=1  orient=off  outDataType=double
  Product : Product  OutDataType=fixdt(1, 16)  OutScaling=2^0  RndMeth=Zero
  Saturation : Saturate  UpperLimit=inf  LowerLimit=0  OutDataType=sfix(16)  OutScaling=2^0
  v_S : Outport  OutDataType=sfix(16)  OutScaling=2^0
  s_S : Outport  Port=2  OutDataType=sfix(16)  OutScaling=2^0
  wires:
  ADC/1 -> s_S/1
  Add/1 -> ADC/1
  Gain/1 -> Add/1
  Gaussian Noise Generator/1 -> Add/2
  Constant/1 -> Dot Product/1, v_S/1
  Saturation/1 -> Gain/1
  v_Sunb/1 -> Dot Product/2
  Dot Product/1 -> Product/1
  Product/1 -> Saturation/1
  light/1 -> Product/2

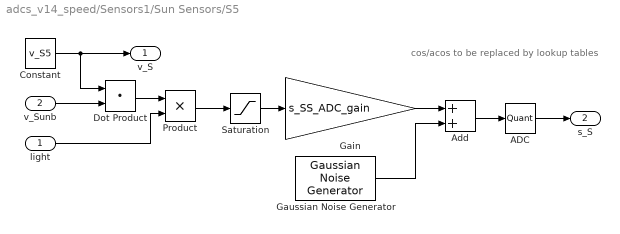
== system adcs_v14_speed/Sensors1/Sun Sensors/S5 ==
  note: cos/acos to be replaced by lookup tables
  light : Inport  OutDataType=sfix(16)  OutScaling=2^0
  v_Sunb : Inport  Port=2  OutDataType=sfix(16)  OutScaling=2^0
  ADC : Quantizer  QuantizationInterval=1/s_SS_ADC_res
  Add : Sum  OutDataType=sfix(16)  OutScaling=2^-10
  Constant : Constant  Value=v_S5  OutDataType=sfix(16)  OutScaling=2^0
  Dot Product : DotProduct  OutDataType=sfix(16)  OutScaling=2^-10  InputSameDT=on  OutDataTypeStr=Inherit: Inherit via internal rule
  Gain : Gain  Gain=s_SS_ADC_gain  ParameterDataType=sfix(16)  ParameterScaling=2^0  OutDataType=sfix(16)  OutScaling=2^0
  Gaussian Noise Generator : commnoisgen2/Gaussian Noise Generator  SystemSampleTime=-1  m=0  d=s_x_SUNSENSOR  s=41  Ts=s_SIM_STEP_SIZE  frameBased=off  sampPerFrame=1  orient=off  outDataType=double
  Product : Product  OutDataType=fixdt(1, 16)  OutScaling=2^0  RndMeth=Zero
  Saturation : Saturate  UpperLimit=inf  LowerLimit=0  OutDataType=sfix(16)  OutScaling=2^0
  v_S : Outport  OutDataType=sfix(16)  OutScaling=2^0
  s_S : Outport  Port=2  OutDataType=sfix(16)  OutScaling=2^0
  wires:
  light/1 -> Product/2
  Product/1 -> Saturation/1
  Dot Product/1 -> Product/1
  v_Sunb/1 -> Dot Product/2
  Saturation/1 -> Gain/1
  Constant/1 -> v_S/1, Dot Product/1
  Gaussian Noise Generator/1 -> Add/2
  Gain/1 -> Add/1
  Add/1 -> ADC/1
  ADC/1 -> s_S/1

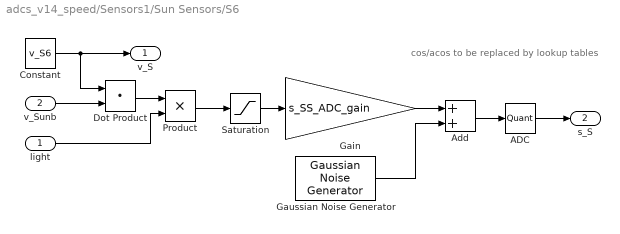
== system adcs_v14_speed/Sensors1/Sun Sensors/S6 ==
  note: cos/acos to be replaced by lookup tables
  light : Inport  OutDataType=sfix(16)  OutScaling=2^0
  v_Sunb : Inport  Port=2  OutDataType=sfix(16)  OutScaling=2^0
  ADC : Quantizer  QuantizationInterval=1/s_SS_ADC_res
  Add : Sum  OutDataType=sfix(16)  OutScaling=2^-10
  Constant : Constant  Value=v_S6  OutDataType=sfix(16)  OutScaling=2^0
  Dot Product : DotProduct  OutDataType=sfix(16)  OutScaling=2^-10  InputSameDT=on  OutDataTypeStr=Inherit: Inherit via internal rule
  Gain : Gain  Gain=s_SS_ADC_gain  ParameterDataType=sfix(16)  ParameterScaling=2^0  OutDataType=sfix(16)  OutScaling=2^0
  Gaussian Noise Generator : commnoisgen2/Gaussian Noise Generator  SystemSampleTime=-1  m=0  d=s_x_SUNSENSOR  s=41  Ts=s_SIM_STEP_SIZE  frameBased=off  sampPerFrame=1  orient=off  outDataType=double
  Product : Product  OutDataType=fixdt(1, 16)  OutScaling=2^0  RndMeth=Zero
  Saturation : Saturate  UpperLimit=inf  LowerLimit=0  OutDataType=sfix(16)  OutScaling=2^0
  v_S : Outport  OutDataType=sfix(16)  OutScaling=2^0
  s_S : Outport  Port=2  OutDataType=sfix(16)  OutScaling=2^0
  wires:
  ADC/1 -> s_S/1
  Add/1 -> ADC/1
  Gain/1 -> Add/1
  Gaussian Noise Generator/1 -> Add/2
  Constant/1 -> Dot Product/1, v_S/1
  Saturation/1 -> Gain/1
  v_Sunb/1 -> Dot Product/2
  Dot Product/1 -> Product/1
  Product/1 -> Saturation/1
  light/1 -> Product/2

== matlab function Torquer/Embedded MATLAB Function4 ==
  data: euler input double; DCM output double
function DCM  = f(euler)
% This block supports the Embedded MATLAB subset.
% See the help menu for details. 

roll = euler(1);
pitch = euler(2);
yaw = euler(3);

rot_x = [  1         0           0;...
             0         cos(roll)  sin(roll);...
             0        -sin(roll)  cos(roll)];
         
rot_y = [cos(pitch)   0       -sin(pitch);...
            0           1        0;...
           sin(pitch)   0        cos(pitch)];
       
rot_z = [ cos(yaw) sin(yaw) 0;...
           -sin(yaw) cos(yaw) 0;...
            0        0            1];
         
DCM  = rot_z *  rot_y *  rot_x;

== matlab function Embedded MATLAB Function ==
  data: x input double; u input double; xdot output double; m_INERTIA parameter double
function xdot = fcn(x, u, m_INERTIA)
% This block supports the Embedded MATLAB subset.
% See the help menu for details. 

q = x(1:4);
w = x(5:7);

W = ...
    [ 0 w(3) -w(2) w(1);
      -w(3) 0 w(1) w(2);
      w(2) -w(1) 0 w(3);
      -w(1) -w(2) -w(3) 0];
  
  qdot = 0.5 * W * q;
  wdot = inv(m_INERTIA)*( u - cross( w, m_INERTIA*w ) );
  
  xdot = [qdot; wdot];

== matlab function Subsystem/f: I->B ==
  data: x input double; v_B output double; v_I input double
function v_B = fcn(x, v_I)
% This block supports the Embedded MATLAB subset.
% See the help menu for details. 

q = x(1:4);

q0 = q(4); q1 = q(1); q2 = q(2); q3 = q(3);

TBI = [ q0^2 + q1^2 - q2^2 - q3^2,         2*q0*q3 + 2*q1*q2,         2*q1*q3 - 2*q0*q2;
           2*q1*q2 - 2*q0*q3, q0^2 - q1^2 + q2^2 - q3^2,         2*q0*q1 + 2*q2*q3;
           2*q0*q2 + 2*q1*q3,         2*q2*q3 - 2*q0*q1, q0^2 - q1^2 - q2^2 + q3^2];

v_B =  TBI*v_I;
v_B = v_B/sqrt(dot(v_B,v_B));

== matlab function I -> B/L_Inertial ==
  data: x input double; v_B output double; v_I input double
function v_B = fcn(x, v_I)
% This block supports the Embedded MATLAB subset.
% See the help menu for details. 

q = x(1:4);

q0 = q(4); q1 = q(1); q2 = q(2); q3 = q(3);

TBI = [ q0^2 + q1^2 - q2^2 - q3^2,         2*q0*q3 + 2*q1*q2,         2*q1*q3 - 2*q0*q2;
           2*q1*q2 - 2*q0*q3, q0^2 - q1^2 + q2^2 - q3^2,         2*q0*q1 + 2*q2*q3;
           2*q0*q2 + 2*q1*q3,         2*q2*q3 - 2*q0*q1, q0^2 - q1^2 - q2^2 + q3^2];

v_B =  TBI*v_I;

== matlab function q -> w/Subsystem6/(1-L) + L/z ==
  data: a input double; y output double; b input double
function y = fcn(a,b)
%#eml

c = 1-a;

y = c+b;
if y>1
    y=1;
end

== matlab function q-normalise ==
  data: x input double; xN output double
function xN  = fcn(x)
% This block gives DCM for converting from ECI to ORBIT frames
% inputs: state vector in ECI
% output: DCM

q = x(1:4);
q = q/sqrt(dot(q,q));
xN = [q; x(5:7)];

== matlab function External Torques/Subsystem/Solar_drag ==
  data: v_Sun_b input double; solar_drag output double; Ca_Solar_Drag parameter double; P_momentum_flux_from_the_sun parameter double; light input double; side parameter double
function solar_drag = fcn(v_Sun_b,Ca_Solar_Drag,P_momentum_flux_from_the_sun,light, side)
% This block supports the Embedded MATLAB subset.
% See the help menu for details. 

% dot product of area vector and sun vector
if (norm(v_Sun_b) == 0)
    u = [1;0;0];
else
    u = v_Sun_b / norm(v_Sun_b);
end

y = 0 ;
a = side;
a = a*a; %Area of satellite
b =  zeros(3,6);
b(:,1) = a*[1;0;0];
b(:,2) = a*[0;1;0];
b(:,3) = a*[0;0;1];
b(:,4) = a*[-1;0;0];
b(:,5) = a*[0;-1;0];
b(:,6) = a*[0;0;-1];

x = 0;
for i=1:6
     x = dot(b(:,i),u);
    if(x>0)
            y = y+x;
    end
end
Ap = y;

solar_drag = -Ap * Ca_Solar_Drag * P_momentum_flux_from_the_sun * u * light;

== matlab function External Torques/L_Inertial ==
  data: x input double; tau output double; v_Si input double; mu parameter double; m_INERTIA parameter double
function tau = fcn(x, v_Si, mu, m_INERTIA)
% This block supports the Embedded MATLAB subset.
% See the help menu for details. 

q = x(1:4);

q0 = q(4); q1 = q(1); q2 = q(2); q3 = q(3);

TBI = [ q0^2 + q1^2 - q2^2 - q3^2,         2*q0*q3 + 2*q1*q2,         2*q1*q3 - 2*q0*q2;
           2*q1*q2 - 2*q0*q3, q0^2 - q1^2 + q2^2 - q3^2,         2*q0*q1 + 2*q2*q3;
           2*q0*q2 + 2*q1*q3,         2*q2*q3 - 2*q0*q1, q0^2 - q1^2 - q2^2 + q3^2];

r_I = v_Si(1:3);
r_B =  TBI*r_I;

R = sqrt(dot(r_B, r_B));
tau = 3*mu * cross( r_B, m_INERTIA*r_B) / R^5;

== matlab function Control Law/q->w ==
  data: B output double; B_l input double; B_k input double; dB output double; s_FRAME_SIZE parameter double
function [B, dB] = fcn(B_l, B_k, s_FRAME_SIZE)
% This block supports the Embedded MATLAB subset.
% See the help menu for details. 

dB = (B_l - B_k)/s_FRAME_SIZE;
B = (B_l + B_k)/2;

== matlab function QuEST ==
  data: v_Bb_m input double; m_SUN input double; q_BO_est output double; v_Bo_c input double; v_So_c input double; s_SS_ADC_gain parameter double; Snum parameter double; light_est output double; s_MAGMETER_WEIGHT parameter double; s_SS_MAX_ANGLE parameter double; v_Sun1 output double
function [q_BO_est, light_est, v_Sun1] = QuEST(v_Bb_m,m_SUN,v_Bo_c,v_So_c, s_SS_ADC_gain, Snum, s_MAGMETER_WEIGHT, s_SS_MAX_ANGLE)

    % Help
    % q_triad = Estimated quaternion
    % b1,b2 = the 2 measurement vectors in body frames
    % r1,r2 = the 2 measurement vectors in reference frames (orbit/inertial; orbit used)
    % b1 is the measurement with very high accurace as compared to b2
    % I am not sure how r1 and r2 will be determined
    % a1 and a2 are Relative weights of b1 and b2


%%%%% calculate v_Sb_m from m_SUN %%%%
t_S = ones(1,Snum)*cos(s_SS_MAX_ANGLE *pi/180);
m_SUN(4,:) = 1.0*(m_SUN(5,:)>t_S);     % set flags from measured voltages

values = m_SUN(5,:);

n_SS = 0;
for i=1:Snum
    if values(i) < 0.5*s_SS_ADC_gain
        n_SS = n_SS + 1;
    end
end

if (n_SS == Snum) 
    light = 0;
else
    light = 1;
end

light_est = light;
%v_Sun1 = [1;0;0];

if (light == 1)    
    
    %%% CALCULATE SUN VECTOR %%%
    
    ssvectors = zeros(3); ssvalues = zeros(3,1); ssflags = zeros(3,1);
     % flags = m_SUN(4,:)';
%     for i=1:3
%         [~, index] = sort(m_SUN(5,:));  % sort values in ascending order
%         z = index(Snum);
%         ssvectors(i,1:3) = m_SUN(1:3,z)';
%         ssflags(i) = m_SUN(4,z);
%         ssvalues(i) = m_SUN(5,z);
%         m_SUN(5,z) = -100 ;
%         for j= 1:Snum
%             if( norm(ssvectors(i,1:3)+m_SUN(1:3,j)') == 0 )
%                 m_SUN(5,j) = -100;
%             end
%         end
%     end
    
    [~, index] = sort(m_SUN(5,:));  % sort values in ascending order
    z = index(Snum); p = 0; % first vector
    ssvectors(1,1:3) = m_SUN(1:3,z)';
    ssvalues(1) = m_SUN(5,z);
    p = p+1;
    
    z = index(Snum-p);  % second vector
    while norm(m_SUN(1:3,z)' + ssvectors(1,1:3)) == 0
        p = p+1;
        z = index(Snum - p);
    end
    ssvectors(2,1:3) = m_SUN(1:3,z)';
    ssvalues(2) = m_SUN(5,z);
    p = p+1;
    
    z = index(Snum-p);  % 3rd vector
    while (norm(m_SUN(1:3,z)' + ssvectors(1,1:3)) == 0) || (norm(m_SUN(1:3,z)' + ssvectors(2,1:3)) == 0)
        p = p+1;
        z = index(Snum - p);
    end
    ssvectors(3,1:3) = m_SUN(1:3,z)';
    ssvalues(3) = m_SUN(5,z);
%     p = p+1;
    
    % v_Sun1 = inv(ssvectors)*ssvalues;
    v_Sun1 = ssvectors\ssvalues;
    v_Sun1 = v_Sun1/sqrt(dot(v_Sun1, v_Sun1));
    v_Sb_m = v_Sun1/sqrt(dot(v_Sun1, v_Sun1));
    
    %%%% start TRIAD %%%%

    b1 = v_Bb_m;
    b2 = v_Sb_m;
    r1 = v_Bo_c;
    r2 = v_So_c;

    a1 = s_MAGMETER_WEIGHT;
    a2 = 1-a1;

    %b3
    b3 = cross(b1,b2);
    b3 = b3/norm(b3) ;
    %r3
    r3 = cross(r1,r2);
    r3 = r3/norm(r3) ;

    %mu
    mu = ( 1 + dot(b3,r3) ) * ( a1*dot(b1,r1) + a2*dot(b2,r2) ) ;
    mu =  mu + dot( cross(b3,r3) , ( a1*cross(b1,r1) + a2*cross(b2,r2) ) ) ;

    %nu
    nu = dot( ( b3 + r3 ) , ( a1*cross(b1,r1) + a2*cross(b2,r2) )  ) ;

    %rho
    rho = sqrt( mu*mu + nu*nu );

    %q
    if( mu > 0)
        k_q_triad = (1/( 2*sqrt( rho*(rho+mu)*( 1 + dot(b3,r3) ) ) ) );
        v_q_triad = ( rho + mu )*( cross(b3,r3) ) + nu*(b3 + r3) ;
        s_q_triad = ( rho + mu )* ( 1 + dot(b3,r3) ) ;
        q_triad = [v_q_triad ; s_q_triad];
        q_triad = k_q_triad * q_triad ;
    else
        k_q_triad = (1/( 2*sqrt( rho*(rho-mu)*( 1 + dot(b3,r3) ) ) ) );
        v_q_triad = ( nu )*( cross(b3,r3) ) + ( rho - mu )*(b3 + r3) ;
        s_q_triad = ( nu )* ( 1 + dot(b3,r3) ) ;
        q_triad = [v_q_triad ; s_q_triad];
        q_triad = k_q_triad * q_triad ;    
    end

    q_triad = q_triad / sqrt(dot(q_triad,q_triad)) ;
    q_BO_est = q_triad;
else
    v_Sun1 = [1 ; 0 ; 0];
    q_BO_est = [0;0;0;1];
    flag_sum = 0;
end
end

== matlab function Satellite Computations I Propagators/m_TOI_NEW1 ==
  data: v_I input double; ECI input double; v_O output double
function v_O  = fcn(v_I, ECI)
% This block gives DCM for converting from ECI to ORBIT frames
% inputs: state vector in ECI
% output: DCM

r = ECI(1:3);   % position vector in ECI
v = ECI(4:6);   % velocity vector in ECI

oy = cross(v,r);    % orbit frame x...
oy = oy/sqrt(dot(oy,oy));

oz = -r/sqrt(dot(r,r));

ox = cross(oy,oz);
ox = ox/sqrt(dot(ox,ox));

TOI = [ox oy oz]';

v_O = TOI*v_I;

== matlab function Control Law/Nominal ==
  data: eu output double; m output double; light input double; w_ctrl input double; w input double; m_N output double; v_B input double; Kp parameter double; Kd parameter double; q input double
function [eu,m,m_N] = fcn(light, w_ctrl, w, v_B, Kp, Kd, q)
% This block supports the Embedded MATLAB subset.
% See the help menu for details. 

Bnorm = sqrt(dot(v_B, v_B));

q = q/sqrt(dot(q,q));

qv = q(1:3);    % e*sin(t/2)
qs = q(4);      %   cos(t/2)

eu = 2*qv*qs;     % 2*e*sin(t/2)*cos(t/2) = e*sin(t)
         
m = (Kp * eu + Kd * w) / Bnorm^2;

m_N = cross( m, v_B ) * light;

== matlab function External Torques/Aerodynamic Torque/aero torque ==
  data: rho input double; v_B input double; u_aero output double; side parameter double; Cd parameter double; v_COM_to_COP_b parameter double
function u_aero = fcn(rho, v_B,side, Cd, v_COM_to_COP_b)

% x = 1;
% z = x*1;
% y = z*u;

% This block supports an embeddable subset of the MATLAB language.
% See the help menu for details. 
% dot product of area vector and velocity vector

vnorm = sqrt(dot(v_B,v_B));
v_unit = v_B / vnorm;

y = 0 ;
a = side;
a = a*a; %Area of satellite
b =  zeros(3,6);
b(:,1) = a*[1;0;0];
b(:,2) = a*[0;1;0];
b(:,3) = a*[0;0;1];
b(:,4) = a*[-1;0;0];
b(:,5) = a*[0;-1;0];
b(:,6) = a*[0;0;-1];

for i=1:6
     x = dot(b(:,i),v_unit);
    if(x>0)
            y = y+x;
    end
end
Ap = y; % total exposed area

F_aero = -0.5 * Cd * rho * Ap * vnorm^2 * v_unit;

u_aero = cross(v_COM_to_COP_b, F_aero);

== matlab function External Torques/Aerodynamic Torque/v_I to v_B ==
  data: v_I input double; x input double; v_B output double
function v_B = fcn(v_I,x)
% This block supports the Embedded MATLAB subset.
% See the help menu for details. 

q = x(1:4);

q0 = q(4); q1 = q(1); q2 = q(2); q3 = q(3);

TBI = [ q0^2 + q1^2 - q2^2 - q3^2,         2*q0*q3 + 2*q1*q2,         2*q1*q3 - 2*q0*q2;
           2*q1*q2 - 2*q0*q3, q0^2 - q1^2 + q2^2 - q3^2,         2*q0*q1 + 2*q2*q3;
           2*q0*q2 + 2*q1*q3,         2*q2*q3 - 2*q0*q1, q0^2 - q1^2 - q2^2 + q3^2];

v_B =  TBI*v_I;

== matlab function Sensors1/Sun Sensors/Embedded MATLAB Function ==
  data: v_S1 input double; m_SUN output double; s_S1 input double; v_S2 input double; s_S2 input double; v_S3 input double; s_S3 input double; v_S4 input double; s_S4 input double; v_S5 input double; s_S5 input double; v_S6 input double; s_S6 input double; Snum parameter double; s_SS_MAX_ANGLE parameter double; values output double
function [m_SUN, values] = fcn(v_S1, s_S1, v_S2, s_S2, v_S3, s_S3, v_S4, s_S4, v_S5, s_S5, v_S6, s_S6, Snum, s_SS_MAX_ANGLE)

a = cos(s_SS_MAX_ANGLE *pi/180);
t_S = ones(1,6)*a;

m_SUNtot = [v_S1 v_S2 v_S3 v_S4 v_S5 v_S6 ; % SS vectors
               0    0    0    0    0    0 ; % flags
            s_S1 s_S2 s_S3 s_S4 s_S5 s_S6 ];% values
        
m_SUNtot(4,:) = 1.0*(m_SUNtot(5,:)>t_S);

m_SUN = m_SUNtot(:, 1:Snum);
values = m_SUN(5,:)';

== matlab function Control Law/Detumbling ==
  data: v_B input double; Bdot input double; Kdetumb parameter double; m_D output double; s_MAG_B parameter double
function m_D = fcn(v_B, Bdot, Kdetumb, s_MAG_B)
% This block supports the Embedded MATLAB subset.
% See the help menu for details. 

Bnorm = sqrt(dot(v_B, v_B));
m_D = -Kdetumb * Bdot * (s_MAG_B / Bnorm);

== matlab function Control Law/Switching Algorithm/gate pulse ==
  data: w input double; q input double; tol_w parameter double; N output double; tol_q4 parameter double; t input double; check_time parameter double; light_flag input double; w_ctrl input double; time1 output double; time2 input double
function [N,time1] = fcn( w, q, tol_w, tol_q4, t,check_time, light_flag, w_ctrl,time2)

modw = sqrt(dot(w, w));
switch_condition = (abs(q(4)) > tol_q4) && (modw < tol_w) && (light_flag ==1) && (w_ctrl == 1);

if (t<100)
    time1=0;
else
    time1=time2;
end

if ( switch_condition )
    N = 1; time1 =t;
elseif (time1==0)
    N=0; time1=0;
elseif (t > (check_time+time1))
    N = 0;
else
    N=1;
end

== matlab function Satellite Computations I Propagators/m_TOI_NEW ==
  data: ECI input double; v_O output double; v_I input double
function v_O  = fcn(ECI, v_I)
% This block gives DCM for converting from ECI to ORBIT frames
% inputs: state vector in ECI
% output: DCM

r = ECI(1:3);   % position vector in ECI
v = ECI(4:6);   % velocity vector in ECI

oy = cross(v,r);    % orbit frame x...
oy = oy/sqrt(dot(oy,oy));

oz = -r/sqrt(dot(r,r));

ox = cross(oy,oz);
ox = ox/sqrt(dot(ox,ox));

TOI = [ox oy oz]';

v_O = TOI*v_I;
